simulink model "lr_disc0"  (R2015a)
settings: Solver=ode45  StartTime=0.0  StopTime=.04  MaxStep=Ts/200  RelTol=1e-3
values from neighbouring files (symbols this model uses):
  alphac = 2*pi*300    (= 1884.95559215)    [Sim_lr_disc0.m]
  L = LAct    (= 0.17)    [Sim_lr_disc0.m]
  R = RAct    (= 3)    [Sim_lr_disc0.m]
  sigmaNoise = 0*.01    (= 0)    [Sim_lr_disc0.m]
  TNoise = Ts    (= 0.0002)    [Sim_lr_disc0.m]
  Ts = 200e-6    (= 0.0002)    [Sim_lr_disc0.m]
  Tsw = 2*Ts    (= 0.0004)    [Sim_lr_disc0.m]
  Udc = 350    [Sim_lr_disc0.m]
  uMax = Udc    (= 350)    [Sim_lr_disc0.m]
undefined symbols (not defined in the file): LAct, RAct
libraries: simulink x2
settings Model: Creator=mhink  LastModifiedBy=mhinkkan
settings DataIOCC: SaveFormat=Dataset
settings HardwareCC: ProdBitPerPointer=64  ProdLargestAtomicFloat=Float  ProdIntDivRoundTo=Zero  ProdEndianess=LittleEndian  ProdHWDeviceType=Specified
settings GRTTargetCC: GeneratePreprocessorConditionals=Use local settings

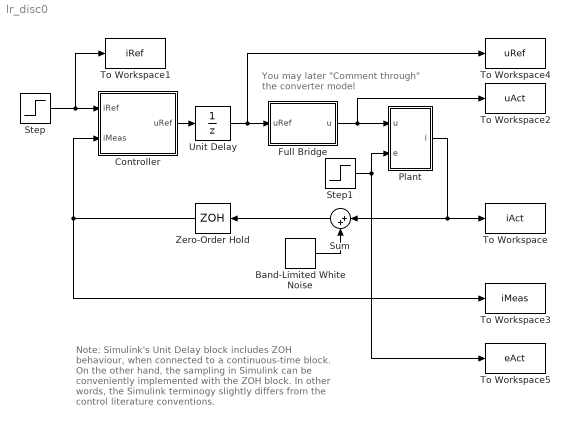
== system lr_disc0 ==
  note: You may later "Comment through"
      | the converter model
  note: Note:
      |
      | Simulink's Unit Delay block includes ZOH behaviour,
      | when connected to a continuous-time block.
      |
      | On the other hand, the sampling in Simulink can be
      | conveniently implemented with the ZOH block.
      |
      | In other words, the Simulink terminogy slightly
      | differs from the control literature conventions.
  Band-Limited White Noise : simulink/Sources/Band-Limited White Noise  Cov=[sigmaNoise^2*TNoise]  Ts=TNoise  seed=[23341]
  Controller : Subsystem
  Full Bridge : Subsystem
  Plant : Subsystem  mask{R=RAct, L=LAct}
      mask prompts: R "Resistance R (ohm)"; L "Inductance L (H)"
  Step : Step  Time=2e-3  After=10  SampleTime=Ts
  Step1 : Step  Time=20e-3  After=100  SampleTime=0
  Sum : Sum  Inputs=|++
  To Workspace : ToWorkspace  VariableName=iAct  SaveFormat=Timeseries  SampleTime=-1
  To Workspace1 : ToWorkspace  VariableName=iRef  SaveFormat=Timeseries  SampleTime=-1
  To Workspace2 : ToWorkspace  VariableName=uAct  SaveFormat=Timeseries  SampleTime=-1
  To Workspace3 : ToWorkspace  VariableName=iMeas  SaveFormat=Timeseries  SampleTime=-1
  To Workspace4 : ToWorkspace  VariableName=uRef  SaveFormat=Timeseries  SampleTime=-1
  To Workspace5 : ToWorkspace  VariableName=eAct  SaveFormat=Timeseries  SampleTime=-1
  Unit Delay : UnitDelay  SampleTime=Ts
  Zero-Order Hold : ZeroOrderHold  SampleTime=Ts
  wires:
  Step/1 -> Controller/1(iRef), To Workspace1/1
  Step1/1 -> Plant/2(e), To Workspace5/1
  Zero-Order Hold/1 -> Controller/2(iMeas), To Workspace3/1
  Controller/1(uRef) -> Unit Delay/1
  Unit Delay/1 -> Full Bridge/1(uRef), To Workspace4/1
  Full Bridge/1(u) -> Plant/1(u), To Workspace2/1
  Plant/1(i) -> To Workspace/1, Sum/1
  Sum/1 -> Zero-Order Hold/1
  Band-Limited White Noise/1 -> Sum/2

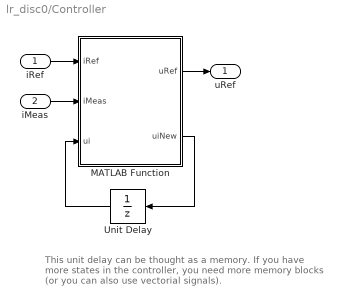
== system lr_disc0/Controller ==
  note: This unit delay can be thought as a memory.
      | If you have more states in the controller, you need more
      | memory blocks (or you can also use vectorial
      | signals).
  iRef : Inport
  iMeas : Inport  Port=2
  MATLAB Function : MATLAB Function  TreatAsAtomicUnit=on
      settings: PermitHierarchicalResolution=ParametersOnly
  Unit Delay : UnitDelay  SampleTime=Ts
  uRef : Outport
  wires:
  Unit Delay/1 -> MATLAB Function/3(ui)
  iRef/1 -> MATLAB Function/1(iRef)
  iMeas/1 -> MATLAB Function/2(iMeas)
  MATLAB Function/1(uRef) -> uRef/1
  MATLAB Function/2(uiNew) -> Unit Delay/1

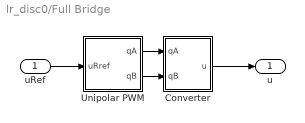
== system lr_disc0/Full Bridge ==
  uRef : Inport
  Converter : Subsystem
  Unipolar PWM : Subsystem
  u : Outport
  wires:
  Converter/1(u) -> u/1
  Unipolar PWM/2(qB) -> Converter/2(qB)
  Unipolar PWM/1(qA) -> Converter/1(qA)
  uRef/1 -> Unipolar PWM/1(uRref)

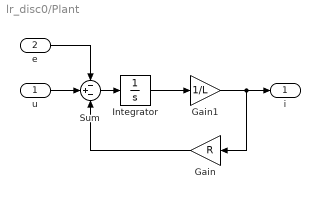
== system lr_disc0/Plant ==
  u : Inport
  e : Inport  Port=2
  Gain : Gain  Gain=R
  Gain1 : Gain  Gain=1/L
  Integrator : Integrator
  Sum : Sum  Inputs=-+-
  i : Outport
  wires:
  u/1 -> Sum/2
  Integrator/1 -> Gain1/1
  Sum/1 -> Integrator/1
  Gain1/1 -> i/1, Gain/1
  e/1 -> Sum/1
  Gain/1 -> Sum/3

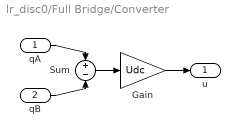
== system lr_disc0/Full Bridge/Converter ==
  qA : Inport
  qB : Inport  Port=2
  Gain : Gain  Gain=Udc
  Sum : Sum  Inputs=+|-
  u : Outport
  wires:
  qA/1 -> Sum/1
  qB/1 -> Sum/2
  Gain/1 -> u/1
  Sum/1 -> Gain/1

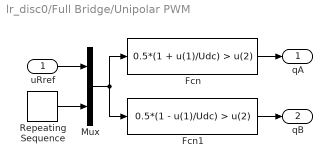
== system lr_disc0/Full Bridge/Unipolar PWM ==
  uRref : Inport
  Fcn : Fcn  Expr=0.5*(1 + u(1)/Udc) > u(2)
  Fcn1 : Fcn  Expr=0.5*(1 - u(1)/Udc) > u(2)
  Mux : Mux  Inputs=2
  Repeating Sequence : simulink/Sources/Repeating Sequence  rep_seq_t=Tsw*[0 0.5 1]  rep_seq_y=[1 0 1]
  qA : Outport
  qB : Outport  Port=2
  wires:
  uRref/1 -> Mux/1
  Mux/1 -> Fcn1/1, Fcn/1
  Repeating Sequence/1 -> Mux/2
  Fcn/1 -> qA/1
  Fcn1/1 -> qB/1

== matlab function lr_disc0/Controller/MATLAB Function ==
  data: uRef output; iRef input; uiNew output; iMeas input; ui input; uMax parameter; alphac parameter; Ts parameter; L parameter; R parameter
function [uRef,uiNew]  = fcn(iRef,iMeas,ui,uMax,alphac,Ts, L, R)

% Note: In order to define the inputs, outputs, and parameters (read from
% workspace), you can press the "Edit Data" button in the ribbon above.

% State feedback, continuous-time design  
kt = alphac*L; k1 = 2*alphac*L - R; ki = Ts*alphac^2*L;  

% Calculate the ideal controller output
uRefIdeal = kt*iRef - k1*iMeas + ui;

% Limit the output
uRef = uRefIdeal;
if(uRef > uMax)
    uRef = uMax;
elseif(uRef < -uMax)
    uRef = -uMax;
end

% Update the integrator state. Last term is the antiwindup.
uiNew = ui + ki*((iRef - iMeas) + (uRef - uRefIdeal)/kt);
